simulink model "quadrotor_v1"  (R2022a)
settings: Solver=VariableStepAuto  StartTime=0.0  StopTime=10.0  RelTol=1e-3
InitFcn:
  | create_vars;
values from neighbouring files (symbols this model uses):
  b = 1    [create_vars.m]
  d = 1    [create_vars.m]
  g = 9.807    [create_vars.m]
  l = 1    [create_vars.m]
  m = 1    [create_vars.m]
libraries: shared6dof x1
settings Model: Creator=Aaron  LastModifiedBy=asoib

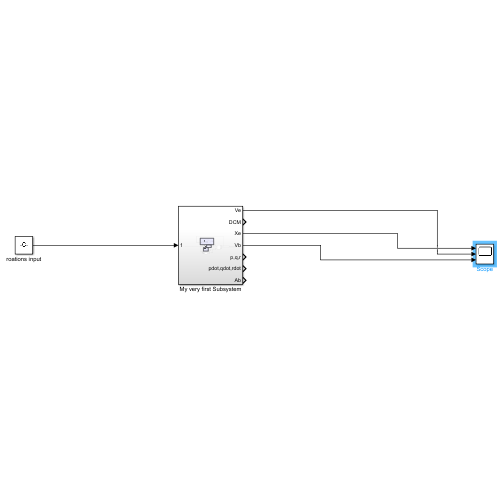
[thumbnail: Simulink's stored preview of the top-level diagram]
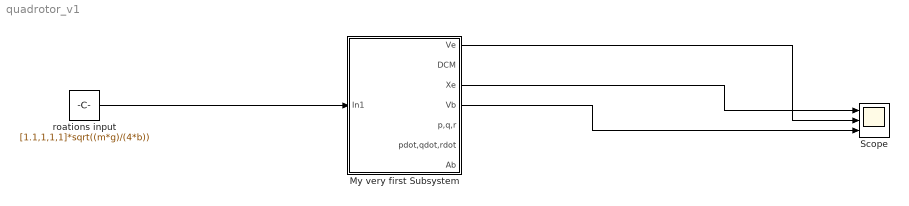
== system quadrotor_v1 ==
  My very first Subsystem : Subsystem
  Scope : Scope  NumInputPorts=3
  roations input : Constant  Value=[1.1,1,1,1]*sqrt((m*g)/(4*b))
  wires:
  roations input/1 -> My very first Subsystem/1(In1)
  My very first Subsystem/3(Xe) -> Scope/1
  My very first Subsystem/4(Vb) -> Scope/3
  My very first Subsystem/1(Ve) -> Scope/2

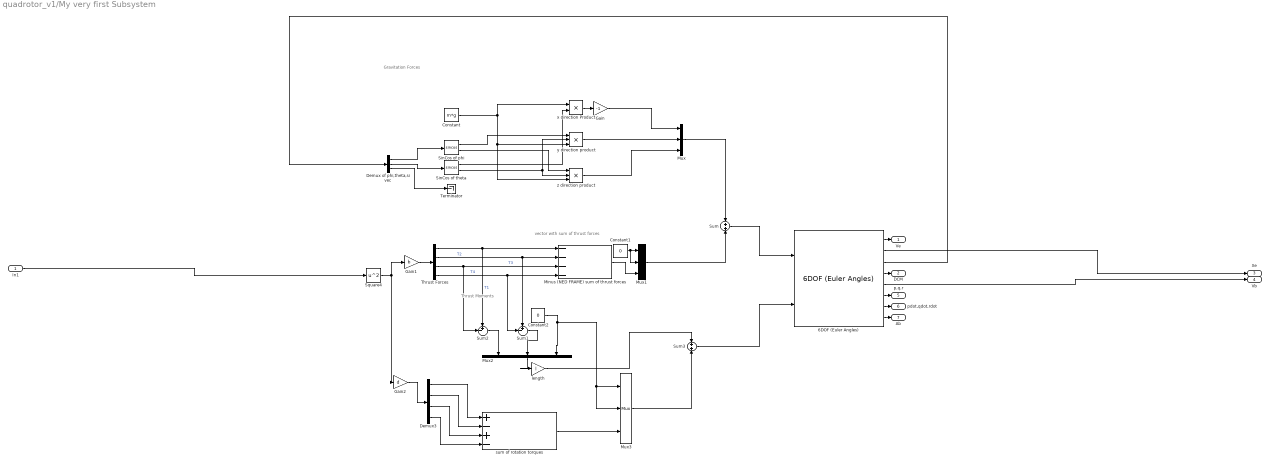
== system quadrotor_v1/My very first Subsystem ==
  note: Thrust Moments
  note: vector with sum of
      | thrust forces
  note: Gravitation Forces
  In1 : Inport
  6DOF (Euler Angles) : shared6dof/6DOF (Euler Angles)  units=Metric (MKS)  mtype=Fixed  rep=Euler Angles  xme_0=[0 0 0]  Vm_0=[0 0 0]  eul_0=[0 0 0]  pm_0=[0 0 0]  mass_0=1.0  mass_e=0.5  mass_f=2.0  inertia=eye(3)  inertia_e=eye(3)  inertia_f=2*eye(3)  k_quat=1.0  vre_flag=on  abi_flag=off  aMode=0  xme_statename=''  Vm_statename=''  eul_statename=''  quat_statename=''  pm_statename=''  mass_statename=''
      settings: SourceProductBaseCode=AE,PW,DR,MT,VE
  Constant : Constant  Value=m*g
  Constant1 : Constant  Value=0
  Constant2 : Constant  Value=0
  Demux of phi,theta,si vec : Demux  Outputs=3
  Demux3 : Demux
  Gain : Gain  Gain=-1
  Gain1 : Gain  Gain=b
  Gain2 : Gain  Gain=d
  Minus (NED FRAME) sum of thrust forces : Sum  Inputs=----
  Mux{,1..3} (4 alike) : Mux  Inputs=3
  SinCos of phi : Trigonometry  Operator=sincos
  SinCos of theta : Trigonometry  Operator=sincos
  Square4 : Math  Operator=square
  Sum : Sum
  Sum1 : Sum  Inputs=+-|
  Sum2 : Sum  Inputs=+-|
  Sum3 : Sum
  Terminator : Terminator
  Thrust Forces : Demux
  length : Gain  Gain=l
  sum of rotation torques : Sum  Inputs=+-+-
  x direction Product : Product
  y direction product : Product  Inputs=3
  z direction product : Product  Inputs=3
  Ve : Outport
  DCM : Outport  Port=2
  Xe : Outport  Port=3
  Vb : Outport  Port=4
  p,q,r : Outport  Port=5
  pdot,qdot,rdot : Outport  Port=6
  Ab : Outport  Port=7
  wires:
  length/1 -> Sum3/1
  Constant1/1 -> Mux1/2, Mux1/1
  Constant/1 -> x direction Product/1, z direction product/3, y direction product/3
  Gain/1 -> Mux/1
  SinCos of phi/2 -> z direction product/1
  Thrust Forces/1 -> Minus (NED FRAME) sum of thrust forces/1, Sum2/1  "T1"
  Sum2/1 -> Mux2/1
  Demux of phi,theta,si vec/1 -> SinCos of phi/1
  6DOF (Euler Angles)/3 -> Demux of phi,theta,si vec/1
  Square4/1 -> Gain1/1, Gain2/1
  sum of rotation torques/1 -> Mux3/3
  Demux3/2 -> sum of rotation torques/2
  Demux of phi,theta,si vec/2 -> SinCos of theta/1
  SinCos of phi/1 -> y direction product/1
  Gain1/1 -> Thrust Forces/1
  6DOF (Euler Angles)/6 -> p,q,r/1
  6DOF (Euler Angles)/1 -> Ve/1
  Constant2/1 -> Mux3/1, Mux3/2, Mux2/3
  Demux3/1 -> sum of rotation torques/1
  Mux2/1 -> length/1
  6DOF (Euler Angles)/7 -> pdot,qdot,rdot/1
  Sum1/1 -> Mux2/2
  6DOF (Euler Angles)/2 -> Xe/1
  Sum3/1 -> 6DOF (Euler Angles)/2
  SinCos of theta/1 -> x direction Product/2
  SinCos of theta/2 -> z direction product/2, y direction product/2
  Demux of phi,theta,si vec/3 -> Terminator/1
  6DOF (Euler Angles)/5 -> Vb/1
  z direction product/1 -> Mux/3
  Demux3/3 -> sum of rotation torques/3
  y direction product/1 -> Mux/2
  Gain2/1 -> Demux3/1
  Demux3/4 -> sum of rotation torques/4
  Thrust Forces/4 -> Minus (NED FRAME) sum of thrust forces/4, Sum1/2  "T4"
  6DOF (Euler Angles)/8 -> Ab/1
  Thrust Forces/2 -> Sum1/1, Minus (NED FRAME) sum of thrust forces/2  "T2"
  Mux3/1 -> Sum3/2
  x direction Product/1 -> Gain/1
  Sum/1 -> 6DOF (Euler Angles)/1
  Mux1/1 -> Sum/2
  Minus (NED FRAME) sum of thrust forces/1 -> Mux1/3
  Mux/1 -> Sum/1
  Thrust Forces/3 -> Minus (NED FRAME) sum of thrust forces/3, Sum2/2  "T3"
  6DOF (Euler Angles)/4 -> DCM/1
  In1/1 -> Square4/1
